simulink model "MDCC"  (R2021b)
settings: Solver=FixedStepDiscrete  StartTime=0.0  StopTime=10.0  FixedStep=0.0001  RelTol=1e-3
model workspace (MATLAB code in the model file):
  | cmdLim = Simulink.Parameter;
  | cmdLim.Value = 15;
  | cmdLim.Description = 'Limit for controlling the maximum surface command angle.';
  | cmdLim.Min = 0;
  | cmdLim.Max = 90;
  | cmdLim.DocUnits = 'deg';
  | 
  | dispGain = Simulink.Parameter;
  | dispGain.Value = 0.75;
  | dispGain.Description = 'Gain applied to the displacement error.';
  | dispGain.Min = 0;
  | dispGain.Max = [];
  | dispGain.DocUnits = 'deg/sec/deg';
  | 
  | dispLim = Simulink.Parameter;
  | dispLim.Value = 30;
  | dispLim.Description = 'Limit for controlling the maximum commanded angle.';
  | dispLim.Min = 0;
  | dispLim.Max = 180;
  | dispLim.DocUnits = 'deg';
  | 
  | intGain = Simulink.Parameter;
  | intGain.Value = 0.5;
  | intGain.Description = 'Gain applied to the integral error.';
  | intGain.Min = 0;
  | intGain.Max = [];
  | intGain.DocUnits = 'deg/sec/deg/sec';
  | 
  | intLim = Simulink.Parameter;
  | intLim.Value = 5;
  | intLim.Description = 'Limit for controlling the maximum commanded angle.';
  | intLim.Min = 0;
  | intLim.Max = 90;
  | intLim.DocUnits = 'deg';
  | 
  | rateGain = Simulink.Parameter;
  | rateGain.Value = 2;
  | rateGain.Description = 'Gain applied to the rate error.';
  | rateGain.Min = 0;
  | rateGain.Max = [];
  | rateGain.DocUnits = 'deg/deg/sec';
  | 
  | rateLim = Simulink.Parameter;
  | rateLim.Value = 6;
  | rateLim.Description = 'Limit for controlling the maximum commanded angle.';
  | rateLim.Min = 0;
  | rateLim.Max = 180;
  | rateLim.DocUnits = 'deg/sec';
  | 
  | hdgGain = Simulink.Parameter;
  | hdgGain.Value = 0.015;
values from neighbouring files (symbols this model uses):
  KfDeadCompen_SetDeltaTime_us = myPackage.Parameter    [DeadCompen.m]
  Ts = 5E-6    (= 5e-06)    [iPMSM_data.m]
  VbDeadComp_SwtUseIsttrDes_flg = myPackage.Parameter    [DeadCompen.m]
  VfDeadCompen_ISttrDdeThdSwt_A = myPackage.Parameter    [DeadCompen.m]
  VfDeadCompen_ISttrIgbtThdSwt_A = myPackage.Parameter    [DeadCompen.m]
  VfDeadCompen_rDdeISttrHi_R = myPackage.Parameter    [DeadCompen.m]
  VfDeadCompen_rDdeISttrLo_R = myPackage.Parameter    [DeadCompen.m]
  VfDeadCompen_rIgbtISttrHi_R = myPackage.Parameter    [DeadCompen.m]
  VfDeadCompen_rIgbtISttrLo_R = myPackage.Parameter    [DeadCompen.m]
  VfDeadCompen_uDdeISttrHi_V = myPackage.Parameter    [DeadCompen.m]
  VfDeadCompen_uDdeISttrLo_V = myPackage.Parameter    [DeadCompen.m]
  VfDeadCompen_uIgbtISttrHi_V = myPackage.Parameter    [DeadCompen.m]
  VfDeadCompen_uIgbtISttrLo_V = myPackage.Parameter    [DeadCompen.m]
undefined symbols (not defined in the file or in its folder): CosTable12bit_Y, GLBCal_GLBCal_Kf_DCLinkOverVolErrThd_V, GLBCal_GLBCal_Kf_DCLinkUnderVolErrThd_V, GLBCal_GLBCal_Kf_EquiLd_NULL, GLBCal_GLBCal_Kf_EquiLq_NULL, GLBCal_GLBCal_Kf_MotorRatedSpeed_rpm, GLBCal_GLBCal_Kf_MotorSpeedHysteresis_Coef, GLBCal_Ke_MotorPolePairsNum_NULL, IoHwAbOpArg_PwmDutyCyclePhU_NULL, IoHwAbOpArg_PwmDutyCyclePhV_NULL, IoHwAbOpArg_PwmDutyCyclePhW_NULL, IoHwAbOpArg_PwmOutputEn, KbMDCC_DeadTimeCompEn_flg, KbMDCC_MCF_flgHarmInIsdqTab11ZR_flg, KbMDCC_MCF_flgHarmInIsdqTab13ZR_flg, KbMDCC_MCF_flgHarmInIsdqTab5ZR_flg, KbMDCC_MCF_flgHarmInIsdqTab7ZR_flg, KbMDCC_MCF_flgHarmInject_flg, KbMDCC_SetEAngleEn_flg, KbMDCC_UdUqFwOmit_flg, KfDeadCompen_CpPeriodTimesT_NULL, KfMDCC_ActiveDischargeIdCurVal_A, KfMDCC_ActiveDischargeIqCurVal_A, KfMDCC_DCLinkVolRate_coef, KfMDCC_DebugEAngleInit_rad, KfMDCC_DebugUalphaVolCmd_V, KfMDCC_DebugUbetaVolCmd_V, KfMDCC_DebugUdCmd_V, KfMDCC_DebugUqCmd_V, KfMDCC_DebugUsCmd_V, KfMDCC_DebugUsRate_V, KfMDCC_IMCResp_NULL, KfMDCC_IMCStab_NULL, KfMDCC_InvParkCpPeriodTimesT_NULL, KfMDCC_MCF_CircAge_NULL, KfMDCC_MCF_flgUse11Harm_flg, KfMDCC_MCF_flgUse13Harm_flg, KfMDCC_MCF_flgUse5Harm_flg, KfMDCC_MCF_flgUse7Harm_flg, KfMDCC_MCF_Harm1113FLParamSpeedThrd_rads, KfMDCC_MCF_Harm57FLParamSpeedThrd_rads, KfMDCC_MCF_HarmcofFltN_NULL, KfMDCC_MCF_HarmCpnAg_NULL, KfMDCC_MCF_HarmfLParaHigh_coef, KfMDCC_MCF_HarmfLParaLow_coef, KfMDCC_MCF_HarmIn1113ZRY_Trq_Nm, KfMDCC_MCF_HarmIn11_SpdLimHigh_rads, KfMDCC_MCF_HarmIn11_SpdLimLow_rads, KfMDCC_MCF_HarmIn11ZRY_Isd_A, KfMDCC_MCF_HarmIn11ZRY_Isq_A, KfMDCC_MCF_HarmIn13_SpdLimHigh_rads, KfMDCC_MCF_HarmIn13_SpdLimLow_rads, KfMDCC_MCF_HarmIn13ZRY_Isd_A, KfMDCC_MCF_HarmIn13ZRY_Isq_A, KfMDCC_MCF_HarmIn57ZRY_Trq_Nm, KfMDCC_MCF_HarmIn5_SpdLimHigh_rads, KfMDCC_MCF_HarmIn5_SpdLimLow_rads, KfMDCC_MCF_HarmIn5ZRY_Isd_A, KfMDCC_MCF_HarmIn5ZRY_Isq_A, KfMDCC_MCF_HarmIn7_SpdLimHigh_rads ... (+47)
libraries: simulink x40, PMSM_Library x3, mcbcontrolslib x1
(part 3 of 8)

== system MDCC/DoCurCtr_sys/MDCC/SVM_Calc/DeadComp_Sys/DeadDuty_Calc ==
  Bus_DutyCompensate : Inport
  CntSctrIs : Inport  Port=2
  Bus Creator : BusCreator  Inputs=7
  Bus Selector : BusSelector  OutputSignals=PwmDuty_0.uDuty,PwmDuty_1.uDuty,PwmDuty_2.uDuty,PwmDuty_3.uDuty,PwmDuty_4.uDuty,PwmDuty_5.uDuty,PwmDuty_fault.uDuty
  Bus Selector1 : BusSelector  OutputSignals=PwmDuty_1.vDuty,PwmDuty_0.vDuty,PwmDuty_2.vDuty,PwmDuty_3.vDuty,PwmDuty_4.vDuty,PwmDuty_5.vDuty,PwmDuty_fault.vDuty
  Bus Selector2 : BusSelector  OutputSignals=PwmDuty_0.wDuty,PwmDuty_1.wDuty,PwmDuty_2.wDuty,PwmDuty_3.wDuty,PwmDuty_4.wDuty,PwmDuty_5.wDuty,PwmDuty_fault.wDuty
  Merge : Merge  Inputs=7
  Merge1 : Merge  Inputs=7
  Merge2 : Merge  Inputs=7
  Switch Case : SwitchCase  CaseConditions={0,1,2,3,4,5}
  Switch Case Action Subsystem : Subsystem  TreatAsAtomicUnit=on
  Switch Case Action Subsystem1 : Subsystem  TreatAsAtomicUnit=on
  Switch Case Action Subsystem2 : Subsystem  TreatAsAtomicUnit=on
  Switch Case Action Subsystem3 : Subsystem  TreatAsAtomicUnit=on
  Switch Case Action Subsystem4 : Subsystem  TreatAsAtomicUnit=on
  Switch Case Action Subsystem5 : Subsystem  TreatAsAtomicUnit=on
  Switch Case Action Subsystem8 : Subsystem  TreatAsAtomicUnit=on
  VfMDSA_DeadCompPwmDutyCyclePhaseU_NULL : Outport
  VfMDSA_DeadCompPwmDutyCyclePhaseV_NULL : Outport  Port=2
  VfMDSA_DeadCompPwmDutyCyclePhaseW_NULL : Outport  Port=3
  wires:
  CntSctrIs/1 -> Switch Case/1
  Switch Case/1 -> [CASE_0]
  Switch Case/2 -> [CASE_1]
  Switch Case/3 -> [CASE_2]
  Switch Case/4 -> [CASE_3]
  Switch Case/5 -> [CASE_4]
  Switch Case/7 -> [default]
  [CASE_0] -> Switch Case Action Subsystem/Action
  [CASE_1] -> Switch Case Action Subsystem1/Action
  [CASE_2] -> Switch Case Action Subsystem2/Action
  [CASE_3] -> Switch Case Action Subsystem3/Action
  [CASE_4] -> Switch Case Action Subsystem4/Action
  [CASE_5] -> Switch Case Action Subsystem5/Action
  [default] -> Switch Case Action Subsystem8/Action
  Switch Case/6 -> [CASE_5]
  Merge/1 -> VfMDSA_DeadCompPwmDutyCyclePhaseU_NULL/1
  Switch Case Action Subsystem/1(PwmDuty) -> Bus Creator/1  "PwmDuty_0"
  Switch Case Action Subsystem1/1(PwmDuty) -> Bus Creator/2  "PwmDuty_1"
  Switch Case Action Subsystem2/1(PwmDuty) -> Bus Creator/3  "PwmDuty_2"
  Switch Case Action Subsystem3/1(PwmDuty) -> Bus Creator/4  "PwmDuty_3"
  Switch Case Action Subsystem4/1(PwmDuty) -> Bus Creator/5  "PwmDuty_4"
  Switch Case Action Subsystem5/1(PwmDuty) -> Bus Creator/6  "PwmDuty_5"
  Switch Case Action Subsystem8/1(PwmDuty) -> Bus Creator/7  "PwmDuty_fault"
  Merge1/1 -> VfMDSA_DeadCompPwmDutyCyclePhaseV_NULL/1
  Merge2/1 -> VfMDSA_DeadCompPwmDutyCyclePhaseW_NULL/1
  Bus Creator/1 -> Bus Selector2/1, Bus Selector1/1, Bus Selector/1
  Bus Selector/1 -> Merge/1  "<uDuty>"
  Bus Selector/2 -> Merge/2  "<uDuty>"
  Bus Selector/3 -> Merge/3  "<uDuty>"
  Bus Selector/4 -> Merge/4  "<uDuty>"
  Bus Selector/5 -> Merge/5  "<uDuty>"
  Bus Selector/6 -> Merge/6  "<uDuty>"
  Bus Selector/7 -> Merge/7  "<uDuty>"
  Bus Selector1/1 -> Merge1/1  "<vDuty>"
  Bus Selector1/2 -> Merge1/2  "<vDuty>"
  Bus Selector1/3 -> Merge1/3  "<vDuty>"
  Bus Selector1/4 -> Merge1/4  "<vDuty>"
  Bus Selector1/5 -> Merge1/5  "<vDuty>"
  Bus Selector1/6 -> Merge1/6  "<vDuty>"
  Bus Selector1/7 -> Merge1/7  "<vDuty>"
  Bus Selector2/1 -> Merge2/1  "<wDuty>"
  Bus Selector2/2 -> Merge2/2  "<wDuty>"
  Bus Selector2/3 -> Merge2/3  "<wDuty>"
  Bus Selector2/4 -> Merge2/4  "<wDuty>"
  Bus Selector2/5 -> Merge2/5  "<wDuty>"
  Bus Selector2/6 -> Merge2/6  "<wDuty>"
  Bus Selector2/7 -> Merge2/7  "<wDuty>"
  Bus_DutyCompensate/1 -> Switch Case Action Subsystem1/1(Bus_DutyCompensate), Switch Case Action Subsystem2/1(Bus_DutyCompensate), Switch Case Action Subsystem3/1(Bus_DutyCompensate), Switch Case Action Subsystem4/1(Bus_DutyCompensate), Switch Case Action Subsystem5/1(Bus_DutyCompensate), Switch Case Action Subsystem8/1("Bus_DutyCorr "), Switch Case Action Subsystem/1(Bus_DutyCompensate)

== system MDCC/DoCurCtr_sys/MDCC/SVM_Calc/DeadComp_Sys/DeadTime_Calc ==
  U_Phase_Dyc : Inport
  V_Phase_Dyc : Inport  Port=2
  W_Phase_Dyc : Inport  Port=3
  iPhase_U : Inport  Port=4
  iPhase_V : Inport  Port=5
  iPhase_W : Inport  Port=6
  uDcLink : Inport  Port=7
  PwmFreq_Hz : Inport  Port=8
  Bus Creator : BusCreator  Inputs=4
  Bus Creator1 : BusCreator  Inputs=3
  DeadTimeDuty_Calc : Subsystem
  DeltaTimeOnOffDuty_Calc : Subsystem
  Tavon_Calc : Subsystem
  Bus_DutyCompensate : Outport
  wires:
  U_Phase_Dyc/1 -> Bus Creator1/1, Tavon_Calc/1(U_Phase_Dyc)  "DutyPhaseU"
  V_Phase_Dyc/1 -> Bus Creator1/2, Tavon_Calc/2(V_Phase_Dyc)  "DutyPhaseV"
  W_Phase_Dyc/1 -> Bus Creator1/3, Tavon_Calc/3(W_Phase_Dyc)  "DutyPhaseW"
  iPhase_U/1 -> DeltaTimeOnOffDuty_Calc/1(iPhase_U), Tavon_Calc/4(iPhase_U)
  iPhase_V/1 -> DeltaTimeOnOffDuty_Calc/2(iPhase_V), Tavon_Calc/5(iPhase_V)
  iPhase_W/1 -> DeltaTimeOnOffDuty_Calc/3(iPhase_W), Tavon_Calc/6(iPhase_W)
  uDcLink/1 -> Tavon_Calc/7(uDcLink)
  PwmFreq_Hz/1 -> DeadTimeDuty_Calc/1(PwmFreq_Hz), DeltaTimeOnOffDuty_Calc/4(PwmFreq_Hz)
  Tavon_Calc/1(Bus_DutyAvon) -> Bus Creator/2  "Bus_DutyAvon"
  DeltaTimeOnOffDuty_Calc/1(Bus_DeltaTimeOnOffDuty) -> Bus Creator/3  "Bus_DeltaTimeOnOffDuty"
  DeadTimeDuty_Calc/1(DeadTimeDuty_NULL) -> Bus Creator/4  "DeadTimeDuty_NULL"
  Bus Creator/1 -> Bus_DutyCompensate/1  "Bus_DutyCompensate"
  Bus Creator1/1 -> Bus Creator/1  "SVM_DutyPhase"

== system MDCC/DoCurCtr_sys/MDCC/SVM_Calc/MDSA/SVM_PU ==
  Ualpha : Inport
  Ubeta : Inport  Port=2
  Add : Sum  Inputs=+-
  Add1 : Sum  Inputs=+-
  Add2 : Sum  Inputs=+-
  Bus Selector : BusSelector  OutputSignals=Tcm1,Tcm2,Tcm3
  Constant : Constant  OutDataTypeStr=single
  Gain : Gain  Gain=2
  Gain1 : Gain  Gain=2
  Gain2 : Gain  Gain=2
  N_Sector_calc : Subsystem
  Saturation : Saturate  UpperLimit=1  LowerLimit=0
  Saturation1 : Saturate  UpperLimit=1  LowerLimit=0
  Saturation2 : Saturate  UpperLimit=1  LowerLimit=0
  Subsystem : Subsystem
  Subsystem1 : Subsystem
  T1_T2_Calc : Subsystem
  Tcm_Calc : Subsystem
  VfMDSA_PwmDutyCyclePhaseU_NULL : Outport  OutMin=0  OutMax=1
  VfMDSA_PwmDutyCyclePhaseV_NULL : Outport  Port=2  OutMin=0  OutMax=1
  VfMDSA_PwmDutyCyclePhaseW_NULL : Outport  Port=3  OutMin=0  OutMax=1
  wires:
  Ualpha/1 -> Subsystem/1(Ualpha), N_Sector_calc/1(Ualpha)
  Ubeta/1 -> Subsystem/2(Ubeta), N_Sector_calc/2(Ubeta)
  N_Sector_calc/1(N_Sector) -> Tcm_Calc/1(N_Sector), T1_T2_Calc/1(N_Sector)
  Subsystem/1(X) -> T1_T2_Calc/2(X)
  Subsystem/2(Y) -> T1_T2_Calc/3(Y)
  Subsystem/3(Z) -> T1_T2_Calc/4(Z)
  Subsystem1/1(Ta) -> Tcm_Calc/2(Ta)
  Subsystem1/2(Tb) -> Tcm_Calc/3(Tb)
  Subsystem1/3(Tc) -> Tcm_Calc/4(Tc)
  Tcm_Calc/1(Bus_CMP) -> Bus Selector/1
  T1_T2_Calc/1(T1) -> Subsystem1/1(T1)
  T1_T2_Calc/2(T2) -> Subsystem1/2(T2)
  Bus Selector/1 -> Gain/1  "<Tcm1>"
  Bus Selector/2 -> Gain1/1  "<Tcm2>"
  Bus Selector/3 -> Gain2/1  "<Tcm3>"
  Constant/1 -> Add2/1, Add1/1, Add/1
  Gain/1 -> Add/2
  Gain1/1 -> Add1/2
  Gain2/1 -> Add2/2
  Add/1 -> Saturation/1
  Add1/1 -> Saturation1/1
  Add2/1 -> Saturation2/1
  Saturation/1 -> VfMDSA_PwmDutyCyclePhaseU_NULL/1
  Saturation1/1 -> VfMDSA_PwmDutyCyclePhaseV_NULL/1
  Saturation2/1 -> VfMDSA_PwmDutyCyclePhaseW_NULL/1

== system MDCC/DoCurCtr_sys/MDCC/SVM_Calc/MDSA/SVPWM ==
  Ualpha_V : Inport
  Ubeta_V : Inport  Port=2
  Ts : Inport  Port=3
  Vdc : Inport  Port=4
  Bus Creator : BusCreator  Inputs=2
  Bus Creator1 : BusCreator  Inputs=2
  Bus Selector : BusSelector  OutputSignals=signal1,signal2,signal3
  Terminator : Terminator
  vIntp_PWMFOC_CalSec : Subsystem  TreatAsAtomicUnit=on  RTWFcnName=vIntp_PWMFOC_CalSec  RTWFileName=vIntp_PWMFOC_CalSec
      settings: RTWFcnNameOpts=User specified  RTWFileNameOpts=User specified
  vIntp_PWMFOC_CalTriCompValue : Subsystem  TreatAsAtomicUnit=on  RTWFcnName=vIntp_PWMFOC_CalTriCompValue  RTWFileName=vIntp_PWMFOC_CalTriCompValue
      settings: RTWFcnNameOpts=User specified  RTWFileNameOpts=User specified
  VfMDSA_PwmDutyCyclePhaseU_NULL : Outport
  VfMDSA_PwmDutyCyclePhaseV_NULL : Outport  Port=2
  VfMDSA_PwmDutyCyclePhaseW_NULL : Outport  Port=3
  wires:
  Bus Selector/3 -> VfMDSA_PwmDutyCyclePhaseW_NULL/1  "<signal3>"
  Bus Selector/2 -> VfMDSA_PwmDutyCyclePhaseV_NULL/1  "<signal2>"
  Bus Selector/1 -> VfMDSA_PwmDutyCyclePhaseU_NULL/1  "<signal1>"
  vIntp_PWMFOC_CalTriCompValue/1(Bus_CMP) -> Bus Selector/1
  vIntp_PWMFOC_CalSec/2(N_VALUE) -> vIntp_PWMFOC_CalTriCompValue/1(N_VALUE_IN)
  vIntp_PWMFOC_CalSec/1(SecValue) -> Terminator/1
  Bus Creator/1 -> vIntp_PWMFOC_CalTriCompValue/2(Bus_UalphaUbeta), vIntp_PWMFOC_CalSec/1(Bus_UalphaUbeta)
  Ualpha_V/1 -> Bus Creator/1  "Ualpha"
  Ubeta_V/1 -> Bus Creator/2  "Ubeta"
  Ts/1 -> Bus Creator1/1  "Ts"
  Vdc/1 -> Bus Creator1/2  "Vdc"
  Bus Creator1/1 -> vIntp_PWMFOC_CalTriCompValue/3(Bus_Ts_Vdc)

== system MDCC/DoCurCtr_sys/MDCC/Simulink Function/Subsystem/If Action Subsystem ==
  In1 : Inport
  Action Port : ActionPort  ActionPortLabel=if(u1 >= u2)
  Constant : Constant  Value=2*pi  OutDataTypeStr=single
  Subtract : Sum  Inputs=+-
  Out1 : Outport
  wires:
  In1/1 -> Subtract/1
  Constant/1 -> Subtract/2
  Subtract/1 -> Out1/1

== system MDCC/DoCurCtr_sys/MDCC/Simulink Function/Subsystem/If Action Subsystem1 ==
  In1 : Inport
  Action Port : ActionPort  ActionPortLabel=elseif(u1 <0)
  Constant : Constant  Value=2*pi  OutDataTypeStr=single
  Subtract : Sum
  Out1 : Outport
  wires:
  In1/1 -> Subtract/1
  Constant/1 -> Subtract/2
  Subtract/1 -> Out1/1

== system MDCC/DoCurCtr_sys/MDCC/Simulink Function/Subsystem/If Action Subsystem2 ==
  In1 : Inport
  Action Port : ActionPort  ActionPortLabel=else
  Out1 : Outport
  wires:
  In1/1 -> Out1/1

== system MDCC/DoCurCtr_sys/MDCC/UdUqCalc_Sys/MDCC_Inverse_Park_Transform/Do_Inverse_Park_Transform ==
  VfMDCC_UdVal_V : Inport
  VfMDCC_UqVal_V : Inport  Port=2
  VfMDCC_SinEAngleNextPWMValue_NULL : Inport  Port=3
  VfMDCC_CosEAngleNextPWMValue_NULL : Inport  Port=4
  Product{,1..3} (4 alike) : Product  RndMeth=Zero
  Subtract : Sum  Inputs=+-
  Subtract1 : Sum
  VfMDCC_VolCmd_alpha_V : Outport
  VfMDCC_VolCmd_beta_V : Outport  Port=2
  wires:
  VfMDCC_UdVal_V/1 -> Product2/1, Product/1
  Product3/1 -> Subtract1/2
  Product2/1 -> Subtract1/1
  Subtract1/1 -> VfMDCC_VolCmd_beta_V/1
  Subtract/1 -> VfMDCC_VolCmd_alpha_V/1
  Product1/1 -> Subtract/2
  VfMDCC_SinEAngleNextPWMValue_NULL/1 -> Product2/2, Product1/2
  VfMDCC_UqVal_V/1 -> Product1/1, Product3/1
  Product/1 -> Subtract/1
  VfMDCC_CosEAngleNextPWMValue_NULL/1 -> Product3/2, Product/2

== system MDCC/DoCurCtr_sys/MDCC/UdUqCalc_Sys/MDCC_MCF_Sys/Clarke1 ==
  VfMDCC_PhaseUCurHarmonic_A : Inport
  VfMDCC_PhaseVCurHarmonic_A : Inport  Port=2
  VfMDCC_PhaseWCurHarmonic_A : Inport  Port=3
  Constant : Constant  Value=0.57735  OutDataTypeStr=single
  Data Type Conversion : DataTypeConversion  OutDataTypeStr=single
  Product : Product
  Subtract : Sum  Inputs=+-
  VfMDCC_AlphaCurHarmonic_A : Outport
  VfMDCC_BetaCurHarmonic_A : Outport  Port=2
  wires:
  Data Type Conversion/1 -> VfMDCC_AlphaCurHarmonic_A/1
  Product/1 -> VfMDCC_BetaCurHarmonic_A/1
  Constant/1 -> Product/2
  Subtract/1 -> Product/1
  VfMDCC_PhaseWCurHarmonic_A/1 -> Subtract/2
  VfMDCC_PhaseVCurHarmonic_A/1 -> Subtract/1
  VfMDCC_PhaseUCurHarmonic_A/1 -> Data Type Conversion/1

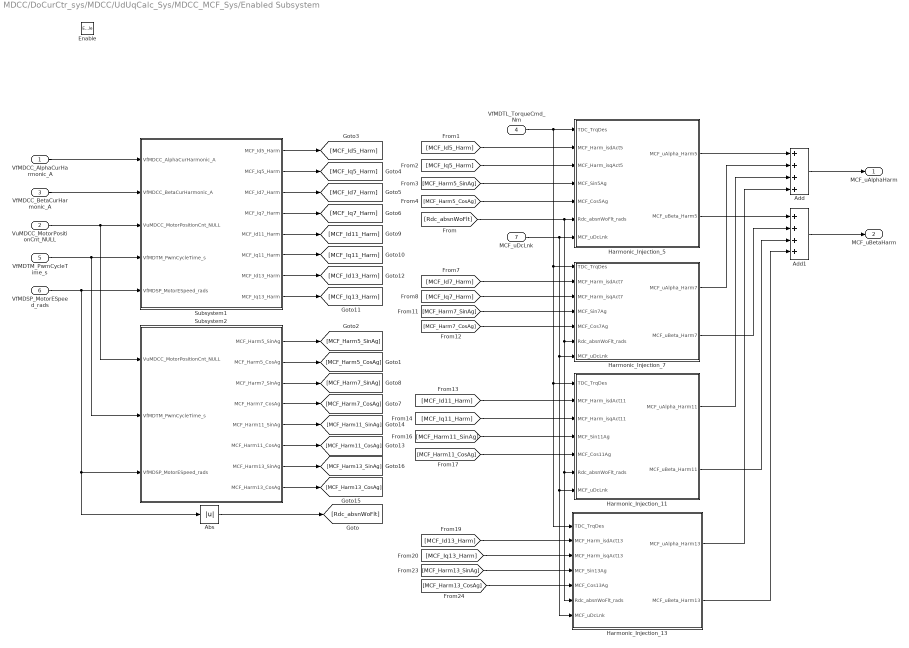
== system MDCC/DoCurCtr_sys/MDCC/UdUqCalc_Sys/MDCC_MCF_Sys/Enabled Subsystem ==
  VfMDCC_AlphaCurHarmonic_A : Inport
  VuMDCC_MotorPositionCnt_NULL : Inport  Port=2
  VfMDCC_BetaCurHarmonic_A : Inport  Port=3
  VfMDTL_TorqueCmd_Nm : Inport  Port=4
  VfMDTM_PwmCycleTime_s : Inport  Port=5
  VfMDSP_MotorESpeed_rads : Inport  Port=6
  MCF_uDcLnk : Inport  Port=7
  Enable : EnablePort
  Abs : Abs
  Add : Sum  Inputs=++++  OutDataTypeStr=single
  Add1 : Sum  Inputs=++++  AccumDataTypeStr=single
  Harmonic_Injection_11 : Subsystem
  Harmonic_Injection_13 : Subsystem
  Harmonic_Injection_5 : Subsystem
  Harmonic_Injection_7 : Subsystem
  Subsystem1 : Subsystem
  Subsystem2 : Subsystem
  MCF_uAlphaHarm : Outport  VectorParamsAs1DForOutWhenUnconnected=off
  MCF_uBetaHarm : Outport  Port=2  VectorParamsAs1DForOutWhenUnconnected=off
  wires:
  VfMDCC_AlphaCurHarmonic_A/1 -> Subsystem1/1(VfMDCC_AlphaCurHarmonic_A)
  VuMDCC_MotorPositionCnt_NULL/1 -> Subsystem2/1(VuMDCC_MotorPositionCnt_NULL), Subsystem1/3(VuMDCC_MotorPositionCnt_NULL)
  VfMDCC_BetaCurHarmonic_A/1 -> Subsystem1/2(VfMDCC_BetaCurHarmonic_A)
  VfMDTM_PwmCycleTime_s/1 -> Subsystem2/2(VfMDTM_PwmCycleTime_s), Subsystem1/4(VfMDTM_PwmCycleTime_s)
  VfMDSP_MotorESpeed_rads/1 -> Abs/1, Subsystem2/3(VfMDSP_MotorESpeed_rads), Subsystem1/5(VfMDSP_MotorESpeed_rads)
  VfMDTL_TorqueCmd_Nm/1 -> Harmonic_Injection_5/1(TDC_TrqDes), Harmonic_Injection_7/1(TDC_TrqDes), Harmonic_Injection_11/1(TDC_TrqDes), Harmonic_Injection_13/1(TDC_TrqDes)
  Subsystem1/1(MCF_Id5_Harm) -> [MCF_Id5_Harm]
  Subsystem1/2(MCF_Iq5_Harm) -> [MCF_Iq5_Harm]
  Subsystem1/3(MCF_Id7_Harm) -> [MCF_Id7_Harm]
  Subsystem1/4(MCF_Iq7_Harm) -> [MCF_Iq7_Harm]
  Subsystem1/5(MCF_Id11_Harm) -> [MCF_Id11_Harm]
  Subsystem1/6(MCF_Iq11_Harm) -> [MCF_Iq11_Harm]
  Subsystem1/7(MCF_Id13_Harm) -> [MCF_Id13_Harm]
  Subsystem1/8(MCF_Iq13_Harm) -> [MCF_Iq13_Harm]
  Subsystem2/1(MCF_Harm5_SinAg) -> [MCF_Harm5_SinAg]
  Subsystem2/2(MCF_Harm5_CosAg) -> [MCF_Harm5_CosAg]
  Subsystem2/3(MCF_Harm7_SinAg) -> [MCF_Harm7_SinAg]
  Subsystem2/4(MCF_Harm7_CosAg) -> [MCF_Harm7_CosAg]
  Subsystem2/5(MCF_Harm11_SinAg) -> [MCF_Harm11_SinAg]
  Subsystem2/6(MCF_Harm11_CosAg) -> [MCF_Harm11_CosAg]
  Subsystem2/7(MCF_Harm13_SinAg) -> [MCF_Harm13_SinAg]
  Subsystem2/8(MCF_Harm13_CosAg) -> [MCF_Harm13_CosAg]
  Abs/1 -> [Rdc_absnWoFlt]
  [MCF_Id5_Harm] -> Harmonic_Injection_5/2(MCF_Harm_isdAct5)
  [MCF_Iq5_Harm] -> Harmonic_Injection_5/3(MCF_Harm_isqAct5)
  [MCF_Harm5_SinAg] -> Harmonic_Injection_5/4(MCF_Sin5Ag)
  [MCF_Harm5_CosAg] -> Harmonic_Injection_5/5(MCF_Cos5Ag)
  [Rdc_absnWoFlt] -> Harmonic_Injection_13/6(Rdc_absnWoFlt_rads), Harmonic_Injection_11/6(Rdc_absnWoFlt_rads), Harmonic_Injection_7/6(Rdc_absnWoFlt_rads), Harmonic_Injection_5/6(Rdc_absnWoFlt_rads)
  MCF_uDcLnk/1 -> Harmonic_Injection_13/7(MCF_uDcLnk), Harmonic_Injection_11/7(MCF_uDcLnk), Harmonic_Injection_7/7(MCF_uDcLnk), Harmonic_Injection_5/7(MCF_uDcLnk)
  [MCF_Id7_Harm] -> Harmonic_Injection_7/2(MCF_Harm_isdAct7)
  [MCF_Iq7_Harm] -> Harmonic_Injection_7/3(MCF_Harm_isqAct7)
  [MCF_Harm7_SinAg] -> Harmonic_Injection_7/4(MCF_Sin7Ag)
  [MCF_Harm7_CosAg] -> Harmonic_Injection_7/5(MCF_Cos7Ag)
  [MCF_Id11_Harm] -> Harmonic_Injection_11/2(MCF_Harm_isdAct11)
  [MCF_Iq11_Harm] -> Harmonic_Injection_11/3(MCF_Harm_isqAct11)
  [MCF_Harm11_SinAg] -> Harmonic_Injection_11/4(MCF_Sin11Ag)
  [MCF_Harm11_CosAg] -> Harmonic_Injection_11/5(MCF_Cos11Ag)
  [MCF_Id13_Harm] -> Harmonic_Injection_13/2(MCF_Harm_isdAct13)
  [MCF_Iq13_Harm] -> Harmonic_Injection_13/3(MCF_Harm_isqAct13)
  [MCF_Harm13_SinAg] -> Harmonic_Injection_13/4(MCF_Sin13Ag)
  [MCF_Harm13_CosAg] -> Harmonic_Injection_13/5(MCF_Cos13Ag)
  Add/1 -> MCF_uAlphaHarm/1
  Harmonic_Injection_5/2(MCF_uBeta_Harm5) -> Add1/1
  Harmonic_Injection_5/1(MCF_uAlpha_Harm5) -> Add/1
  Harmonic_Injection_11/2(MCF_uBeta_Harm11) -> Add1/3
  Add1/1 -> MCF_uBetaHarm/1
  Harmonic_Injection_13/1(MCF_uAlpha_Harm13) -> Add/4
  Harmonic_Injection_7/2(MCF_uBeta_Harm7) -> Add1/2
  Harmonic_Injection_11/1(MCF_uAlpha_Harm11) -> Add/3
  Harmonic_Injection_7/1(MCF_uAlpha_Harm7) -> Add/2
  Harmonic_Injection_13/2(MCF_uBeta_Harm13) -> Add1/4

== system MDCC/DoCurCtr_sys/MDCC/UdUqCalc_Sys/MDCC_MCF_Sys/Subsystem ==
  VfMDSP_PhaseUCurVal_A : Inport  OutDataTypeStr=single
  VfMDSP_PhaseVCurVal_A : Inport  Port=2  OutDataTypeStr=single
  VfMDSP_PhaseWCurVal_A : Inport  Port=3  OutDataTypeStr=single
  VfMDTM_PwmCycleTime_s : Inport  Port=4  OutDataTypeStr=single
  VfMDSP_MotorESpeed_rads : Inport  Port=5  OutDataTypeStr=single
  Add : Sum  Inputs=+-
  Add1 : Sum  Inputs=+-
  Add2 : Sum  Inputs=+-
  iU_SOGI : Subsystem  TreatAsAtomicUnit=on
      settings: RTWSystemCode=Nonreusable function
  iV_SOGI : Subsystem  TreatAsAtomicUnit=on
      settings: RTWSystemCode=Nonreusable function
  iW_SOGI : Subsystem  TreatAsAtomicUnit=on
      settings: RTWSystemCode=Nonreusable function
  VfMDCC_PhaseUCurHarmonic_A : Outport
  VfMDCC_PhaseVCurHarmonic_A : Outport  Port=2
  VfMDCC_PhaseWCurHarmonic_A : Outport  Port=3
  wires:
  iW_SOGI/1(iPhaseBase_A) -> Add2/2
  VfMDSP_PhaseUCurVal_A/1 -> iU_SOGI/1(MCF_iPhase), Add/1
  VfMDSP_MotorESpeed_rads/1 -> iW_SOGI/2(MotorESpeed_rads), iV_SOGI/2(MotorESpeed_rads), iU_SOGI/2(MotorESpeed_rads)
  iU_SOGI/1(iPhaseBase_A) -> Add/2
  VfMDTM_PwmCycleTime_s/1 -> iW_SOGI/3(PwmCycleTime_s), iV_SOGI/3(PwmCycleTime_s), iU_SOGI/3(PwmCycleTime_s)
  VfMDSP_PhaseVCurVal_A/1 -> iV_SOGI/1(MCF_iPhase), Add1/1
  Add1/1 -> VfMDCC_PhaseVCurHarmonic_A/1
  VfMDSP_PhaseWCurVal_A/1 -> iW_SOGI/1(MCF_iPhase), Add2/1
  iV_SOGI/1(iPhaseBase_A) -> Add1/2
  Add/1 -> VfMDCC_PhaseUCurHarmonic_A/1
  Add2/1 -> VfMDCC_PhaseWCurHarmonic_A/1

== system MDCC/DoCurCtr_sys/MDCC/UdUqCalc_Sys/ModDegPwrFacCal/isCal ==
  id : Inport
  iq : Inport  Port=2
  Add : Sum
  Product : Product
  Product1 : Product
  Sqrt : Sqrt  SaturateOnIntegerOverflow=on
  is : Outport
  wires:
  iq/1 -> Product1/2, Product1/1
  id/1 -> Product/2, Product/1
  Product1/1 -> Add/2
  Sqrt/1 -> is/1
  Product/1 -> Add/1
  Add/1 -> Sqrt/1

== system MDCC/DoCurCtr_sys/MDCC/UdUqCalc_Sys/ModDegPwrFacCal/pwrCal ==
  id : Inport
  iq : Inport  Port=2
  ud : Inport  Port=3
  uq : Inport  Port=4
  Add : Sum
  Product : Product
  Product1 : Product
  pwr : Outport
  wires:
  Product/1 -> Add/1
  Product1/1 -> Add/2
  id/1 -> Product/1
  ud/1 -> Product/2
  iq/1 -> Product1/1
  uq/1 -> Product1/2
  Add/1 -> pwr/1

== system MDCC/DoCurCtr_sys/MDCC/UdUqCalc_Sys/ModDegPwrFacCal/usCal ==
  ud : Inport
  uq : Inport  Port=2
  Add : Sum
  Product : Product
  Product1 : Product
  Sqrt : Sqrt  SaturateOnIntegerOverflow=on
  us : Outport
  wires:
  Add/1 -> Sqrt/1
  Product/1 -> Add/1
  Sqrt/1 -> us/1
  Product1/1 -> Add/2
  ud/1 -> Product/1, Product/2
  uq/1 -> Product1/1, Product1/2

== system MDCC/DoCurCtr_sys/MDCC/UdUqCalc_Sys/SelfHeating/Subsystem1 ==
  VfMDTM_SelfHeatingEAngle_NULL : Inport
  VbMDTM_SelfHeatingSinWaveEn_flg : Inport  Port=2
  VbMDSP_McuFSelfheatingMode_flg : Inport  Port=3
  Constant : Constant  Value=uint8(100)
  Constant1 : Constant  Value=KfMDCC_SelfHeatingUdVal_V
  Constant3 : Constant  Value=0  OutDataTypeStr=single
  Constant6 : Constant  Value=KfMDCC_SelfHeatingUdValRate_V
  Merge : Merge
  NOT : Logic  Operator=NOT  IconShape=distinctive  AllPortsSameDT=off  OutDataTypeStr=boolean
  Signal Copy : SignalConversion  OverrideOpt=off
  SinCounter_10ms : Subsystem  TreatAsAtomicUnit=on
      settings: RTWSystemCode=Nonreusable function  RTWFcnNameOpts=Use subsystem name
  Subsystem : Subsystem
  Subsystem1 : Subsystem
  Subsystem2 : Subsystem
  Switch : Switch  Criteria=u2 ~= 0
  VfMDCC_SelfHeatingUdVal_V : Outport
  VbMDCC_SelfHeatingStop_flg : Outport  Port=2
  wires:
  VfMDTM_SelfHeatingEAngle_NULL/1 -> Subsystem2/1(VfMDTM_SelfHeatingEAngle_NULL), Subsystem/1(VfMDTM_SelfHeatingEAngle_NULL)
  VbMDTM_SelfHeatingSinWaveEn_flg/1 -> NOT/1, Subsystem/Enable
  NOT/1 -> Subsystem2/Enable
  Subsystem/1(VfMDTM_SelfHeatingUdVal_V) -> Merge/1
  Subsystem2/1(VfMDTM_SelfHeatingUdVal_V) -> Merge/2
  Merge/1 -> Signal Copy/1  "MDCC_VfMDCC_SelfHeatingUdVal_V"
  Constant6/1 -> Subsystem1/2(rate)
  SinCounter_10ms/1(En) -> Subsystem1/Enable  "En"
  Constant/1 -> SinCounter_10ms/1(CNT)
  Subsystem1/1(VfMDTM_SelfHeatingUdVal_V_Set) -> Subsystem/2(VfMDTM_SelfHeatingUdVal_V_Set), Subsystem2/2(VfMDTM_SelfHeatingUdVal_V_Set)  "VfMDTM_SelfHeatingUdVal_V_Set"
  Subsystem1/2(VbMDCC_SelfHeatingStop_flg) -> VbMDCC_SelfHeatingStop_flg/1
  Constant3/1 -> Switch/3
  Constant1/1 -> Switch/1
  Switch/1 -> Subsystem1/1(set)
  VbMDSP_McuFSelfheatingMode_flg/1 -> Switch/2
  Signal Copy/1 -> VfMDCC_SelfHeatingUdVal_V/1

== system MDCC/DoCurCtr_sys/MDCC/UdUqCalc_Sys/UdUqCalc/IsDQCtl_200us ==
  PIReset : Inport
  TQC_IsdDes : Inport  Port=2
  TQC_IsqDes : Inport  Port=3
  ISM_Isd : Inport  Port=4
  ISM_Isq : Inport  Port=5
  TQC_omSttr : Inport  Port=6
  TQC_dtIsctl_Cc : Inport  Port=7
  TQC_kidq : Inport  Port=8
  TQC_kpd : Inport  Port=9
  TQC_kpq : Inport  Port=10
  TQC_Rv : Inport  Port=11
  TQC_UsqFluxExc : Inport  Port=12
  TQC_uDaMax_Cc : Inport  Port=13
  TQC_uQaMax_Cc : Inport  Port=14
  IsDQCtl_m : MATLAB Function  TreatAsAtomicUnit=on  VariantControl=IsDQCtl_m
      settings: RTWSystemCode=Nonreusable function  RTWFcnNameOpts=Use subsystem name
  TQC_UsdPI : Outport
  TQC_UsqPI : Outport  Port=2
  facIntglDa_Dbg : Outport  Port=3
  facIntglQa_Dbg : Outport  Port=4
  facIntglDaQa_Dbg : Outport  Port=5
  uDaUnlim_Dbg : Outport  Port=6
  uQaUnlim_Dbg : Outport  Port=7
  iDaDes_Dbg : Outport  Port=8
  iQaDes_Dbg : Outport  Port=9

== system MDCC/DoCurCtr_sys/MDCC/UdUqCalc_Sys/UdUqCalc/Subsystem ==
  VfMDSP_MotorAveAbsSpeed_rpm : Inport
  VfMDSP_MotorRs_Ohm : Inport  Port=2
  1-D Lookup Table : Lookup_n-D  NumberOfTableDimensions=1  BreakpointsForDimension1=KfMDCC_SpdIMCResp_rpm  BreakpointsForDimension1DataTypeStr=Inherit: Inherit from 'Breakpoint data'  IndexSearchMethod=Linear search  Table=KfMDCC_IMCResp_NULL  TableDataTypeStr=Inherit: Inherit from 'Table data'  ExtrapMethod=Clip  UseLastTableValue=on  InternalRulePriority=Speed  OutDataTypeStr=Inherit: Inherit from 'Table data'  RndMeth=Simplest
  1-D Lookup Table1 : Lookup_n-D  NumberOfTableDimensions=1  BreakpointsForDimension1=KfMDCC_SpdIMCStab_rpm  BreakpointsForDimension1DataTypeStr=Inherit: Inherit from 'Breakpoint data'  IndexSearchMethod=Linear search  Table=KfMDCC_IMCStab_NULL  TableDataTypeStr=Inherit: Inherit from 'Table data'  ExtrapMethod=Clip  UseLastTableValue=on  InternalRulePriority=Speed  OutDataTypeStr=Inherit: Inherit from 'Table data'  RndMeth=Simplest
  Add : Sum
  Constant : Constant  Value=GLBCal_GLBCal_Kf_EquiLq_NULL
  Constant1 : Constant  Value=GLBCal_GLBCal_Kf_EquiLd_NULL
  Product{,1,4..5} (4 alike) : Product  OutDataTypeStr=single  RndMeth=Round
  VfMDCC_Rv_Ohm : Outport
  KfMDCC_Kidq_NULL : Outport  Port=2
  KfMDCC_Kpd_NULL : Outport  Port=3
  KfMDCC_Kpq_NULL : Outport  Port=4
  wires:
  Product/1 -> VfMDCC_Rv_Ohm/1, Add/1  "VfMDCC_Rv_Ohm"
  VfMDSP_MotorAveAbsSpeed_rpm/1 -> 1-D Lookup Table/1, 1-D Lookup Table1/1
  Constant1/1 -> Product4/2
  [StabAdap] -> Product1/2
  1-D Lookup Table/1 -> [RespScal]  "VfMDCC_RespScal_NULL"
  1-D Lookup Table1/1 -> Product/1
  VfMDSP_MotorRs_Ohm/1 -> Product/2, Add/2
  [RespScal] -> Product4/1
  [RespScal] -> Product5/1
  [RespScal] -> Product1/1
  Constant/1 -> Product5/2
  Product1/1 -> KfMDCC_Kidq_NULL/1  "KfMDCC_Kidq_NULL"
  Add/1 -> [StabAdap]  "VfMDCC_KidqStabAdap_NULL"
  Product5/1 -> KfMDCC_Kpq_NULL/1  "KfMDCC_Kpq_NULL"
  Product4/1 -> KfMDCC_Kpd_NULL/1  "KfMDCC_Kpd_NULL"

== system MDCC/DoCurCtr_sys/MDCC/SVM_Calc/DeadComp_Sys/DeadCur_Calc/Inverse_Clarke_Transform ==
  Alpha : Inport
  Beta : Inport  Port=2
  add_b : Sum  Inputs=-+  RndMeth=Simplest  OutDataTypeStr=Inherit: Same as first input
  add_c : Sum  Inputs=--  RndMeth=Simplest  OutDataTypeStr=Inherit: Same as first input
  one_by_two : Gain  Gain=1/2  RndMeth=Simplest  OutDataTypeStr=Inherit: Same as input
  sqrt3_by_two : Gain  Gain=sqrt(3)/2  RndMeth=Simplest  OutDataTypeStr=Inherit: Same as input
  a : Outport  VectorParamsAs1DForOutWhenUnconnected=off
  b : Outport  Port=2  VectorParamsAs1DForOutWhenUnconnected=off
  c : Outport  Port=3  VectorParamsAs1DForOutWhenUnconnected=off
  wires:
  Beta/1 -> sqrt3_by_two/1
  sqrt3_by_two/1 -> add_c/2, add_b/2
  one_by_two/1 -> add_b/1, add_c/1
  add_c/1 -> c/1
  Alpha/1 -> one_by_two/1, a/1
  add_b/1 -> b/1

== system MDCC/DoCurCtr_sys/MDCC/SVM_Calc/DeadComp_Sys/DeadCur_Calc/IsdqSelect_Calc ==
  IsdDes_A : Inport
  IsqDes_A : Inport  Port=2
  IsdFb_A : Inport  Port=3
  IsqFb_A : Inport  Port=4
  Bus Creator : BusCreator  Inputs=2
  Bus Creator1 : BusCreator  Inputs=2
  Bus Selector : BusSelector  OutputSignals=Isd_A,Isq_A
  Constant : Constant  Value=VbDeadComp_SwtUseIsttrDes_flg
  Switch : Switch  Criteria=u2 ~= 0
  Isd_A : Outport
  Isq_A : Outport  Port=2
  wires:
  Bus Creator1/1 -> Switch/3
  IsqDes_A/1 -> Bus Creator/2  "Isq_A"
  Bus Creator/1 -> Switch/1
  IsqFb_A/1 -> Bus Creator1/2  "Isq_A"
  IsdFb_A/1 -> Bus Creator1/1  "Isd_A"
  Constant/1 -> Switch/2
  IsdDes_A/1 -> Bus Creator/1  "Isd_A"
  Switch/1 -> Bus Selector/1
  Bus Selector/1 -> Isd_A/1  "<Isd_A>"
  Bus Selector/2 -> Isq_A/1  "<Isq_A>"

== system MDCC/DoCurCtr_sys/MDCC/SVM_Calc/DeadComp_Sys/DeadCur_Calc/N_Select_Calc ==
  eMtrSpd_rads : Inport
  eMtrPos_NULL : Inport  Port=2
  VfPwmFreq_Hz : Inport  Port=3
  Isd_A : Inport  Port=4
  Isq_A : Inport  Port=5
  Add : Sum  Inputs=+++
  Constant2 : Constant  Value=2*pi  OutDataTypeStr=single
  Constant3 : Constant  Value=pi/6  OutDataTypeStr=single
  Constant4 : Constant  Value=pi/3  OutDataTypeStr=single
  Data Type Conversion : DataTypeConversion  OutDataTypeStr=uint8
  Data Type Conversion1 : DataTypeConversion  OutDataTypeStr=uint16
  Divide : Product  Inputs=*/
  Gain : Gain  Gain=4095/(2*pi)
  Mod : Math  Operator=mod  SaturateOnIntegerOverflow=on
  Subsystem1 : Subsystem
  Subsystem2 : Subsystem
  PreMtrPos : Outport
  Select_N : Outport  Port=2
  wires:
  Constant3/1 -> Add/3
  Mod/1 -> Divide/1
  Subsystem2/1(PreMtrPos) -> Gain/1, Add/1
  Constant2/1 -> Mod/2
  eMtrPos_NULL/1 -> Subsystem2/2(eMtrPos_NULL)
  Add/1 -> Mod/1
  Subsystem1/1(agIsE) -> Add/2
  Divide/1 -> Data Type Conversion/1
  Constant4/1 -> Divide/2
  Data Type Conversion/1 -> Select_N/1
  Isq_A/1 -> Subsystem1/2(Isq_A)
  Isd_A/1 -> Subsystem1/1(Isd_A)
  VfPwmFreq_Hz/1 -> Subsystem2/3(VfPwmFreq_Hz)
  eMtrSpd_rads/1 -> Subsystem2/1(eMtrSpd_rads)
  Gain/1 -> Data Type Conversion1/1
  Data Type Conversion1/1 -> PreMtrPos/1

== system MDCC/DoCurCtr_sys/MDCC/SVM_Calc/DeadComp_Sys/DeadCur_Calc/SineCosineLookup_Calc ==
  PreMtrPos : Inport
  Cos12bit : LookupNDDirect  NumberOfTableDimensions=1  Table=CosTable12bit_Y  TableDataTypeStr=single
  Sin12bit : LookupNDDirect  NumberOfTableDimensions=1  Table=SinTable12bit_Y  TableDataTypeStr=single
  sin : Outport  VectorParamsAs1DForOutWhenUnconnected=off
  cos : Outport  Port=2  VectorParamsAs1DForOutWhenUnconnected=off
  wires:
  PreMtrPos/1 -> Cos12bit/1, Sin12bit/1
  Cos12bit/1 -> cos/1
  Sin12bit/1 -> sin/1

== system MDCC/DoCurCtr_sys/MDCC/SVM_Calc/DeadComp_Sys/DeadCur_Calc/iPark_Calc ==
  Ds : Inport
  Qs : Inport  Port=2
  sin : Inport  Port=3
  cos : Inport  Port=4
  dcos : Product  RndMeth=Simplest  OutDataTypeStr=Inherit: Same as first input
  dsin : Product  RndMeth=Simplest  OutDataTypeStr=Inherit: Same as first input
  qcos : Product  RndMeth=Simplest  OutDataTypeStr=Inherit: Same as first input
  qsin : Product  RndMeth=Simplest  OutDataTypeStr=Inherit: Same as first input
  sum_alpha : Sum  Inputs=|+-  RndMeth=Simplest  OutDataTypeStr=Inherit: Same as first input
  sum_beta : Sum  Inputs=|++  RndMeth=Simplest  OutDataTypeStr=Inherit: Same as first input
  Alpha : Outport  VectorParamsAs1DForOutWhenUnconnected=off
  Beta : Outport  Port=2  VectorParamsAs1DForOutWhenUnconnected=off
  wires:
  qcos/1 -> sum_beta/1
  Qs/1 -> qsin/1, qcos/1
  dcos/1 -> sum_alpha/1
  sin/1 -> dsin/2, qsin/2
  cos/1 -> qcos/2, dcos/2
  qsin/1 -> sum_alpha/2
  Ds/1 -> dcos/1, dsin/1
  dsin/1 -> sum_beta/2
  sum_beta/1 -> Beta/1
  sum_alpha/1 -> Alpha/1

== system MDCC/DoCurCtr_sys/MDCC/SVM_Calc/DeadComp_Sys/DeadDuty_Calc/Switch Case Action Subsystem ==
  Bus_DutyCompensate : Inport
  Action Port : ActionPort  ActionPortLabel=case [ 0 ]:
  Add : Sum  Inputs=++-
  Add1 : Sum  Inputs=+-+
  Add2 : Sum  Inputs=+-+
  Bus Creator : BusCreator  Inputs=3
  Bus Selector : BusSelector  OutputSignals=Bus_DutyAvon.DeadDutyAvon_U,DeadTimeDuty_NULL,Bus_DeltaTimeOnOffDuty.DeltaTimeOnOffU_NULL
  Bus Selector1 : BusSelector  OutputSignals=Bus_DutyAvon.DeadDutyAvon_V,DeadTimeDuty_NULL,Bus_DeltaTimeOnOffDuty.DeltaTimeOnOffV_NULL
  Bus Selector2 : BusSelector  OutputSignals=Bus_DutyAvon.DeadDutyAvon_W,DeadTimeDuty_NULL,Bus_DeltaTimeOnOffDuty.DeltaTimeOnOffW_NULL
  PwmDuty : Outport
  wires:
  Add/1 -> Bus Creator/1  "uDuty"
  Add1/1 -> Bus Creator/2  "vDuty"
  Add2/1 -> Bus Creator/3  "wDuty"
  Bus Creator/1 -> PwmDuty/1
  Bus_DutyCompensate/1 -> Bus Selector/1, Bus Selector2/1, Bus Selector1/1
  Bus Selector/1 -> Add/1  "<DeadDutyAvon_U>"
  Bus Selector/3 -> Add/3  "<DeltaTimeOnOffU_NULL>"
  Bus Selector1/2 -> Add1/2  "<DeadTimeDuty_NULL>"
  Bus Selector1/1 -> Add1/1  "<DeadDutyAvon_V>"
  Bus Selector2/1 -> Add2/1  "<DeadDutyAvon_W>"
  Bus Selector2/2 -> Add2/2  "<DeadTimeDuty_NULL>"
  Bus Selector/2 -> Add/2  "<DeadTimeDuty_NULL>"
  Bus Selector1/3 -> Add1/3  "<DeltaTimeOnOffV_NULL>"
  Bus Selector2/3 -> Add2/3  "<DeltaTimeOnOffW_NULL>"

== system MDCC/DoCurCtr_sys/MDCC/SVM_Calc/DeadComp_Sys/DeadDuty_Calc/Switch Case Action Subsystem1 ==
  Bus_DutyCompensate : Inport
  Action Port : ActionPort  ActionPortLabel=case [ 1 ]:
  Add : Sum  Inputs=++-
  Add1 : Sum  Inputs=++-
  Add2 : Sum  Inputs=+-+
  Bus Creator : BusCreator  Inputs=3
  Bus Selector : BusSelector  OutputSignals=Bus_DutyAvon.DeadDutyAvon_U,DeadTimeDuty_NULL,Bus_DeltaTimeOnOffDuty.DeltaTimeOnOffU_NULL
  Bus Selector1 : BusSelector  OutputSignals=Bus_DutyAvon.DeadDutyAvon_V,DeadTimeDuty_NULL,Bus_DeltaTimeOnOffDuty.DeltaTimeOnOffV_NULL
  Bus Selector2 : BusSelector  OutputSignals=Bus_DutyAvon.DeadDutyAvon_W,DeadTimeDuty_NULL,Bus_DeltaTimeOnOffDuty.DeltaTimeOnOffW_NULL
  PwmDuty : Outport
  wires:
  Add/1 -> Bus Creator/1  "uDuty"
  Add1/1 -> Bus Creator/2  "vDuty"
  Add2/1 -> Bus Creator/3  "wDuty"
  Bus Creator/1 -> PwmDuty/1
  Bus_DutyCompensate/1 -> Bus Selector/1, Bus Selector2/1, Bus Selector1/1
  Bus Selector/1 -> Add/1  "<DeadDutyAvon_U>"
  Bus Selector/3 -> Add/3  "<DeltaTimeOnOffU_NULL>"
  Bus Selector1/2 -> Add1/2  "<DeadTimeDuty_NULL>"
  Bus Selector1/1 -> Add1/1  "<DeadDutyAvon_V>"
  Bus Selector2/1 -> Add2/1  "<DeadDutyAvon_W>"
  Bus Selector2/2 -> Add2/2  "<DeadTimeDuty_NULL>"
  Bus Selector/2 -> Add/2  "<DeadTimeDuty_NULL>"
  Bus Selector1/3 -> Add1/3  "<DeltaTimeOnOffV_NULL>"
  Bus Selector2/3 -> Add2/3  "<DeltaTimeOnOffW_NULL>"

== system MDCC/DoCurCtr_sys/MDCC/SVM_Calc/DeadComp_Sys/DeadDuty_Calc/Switch Case Action Subsystem2 ==
  Bus_DutyCompensate : Inport
  Action Port : ActionPort  ActionPortLabel=case [ 2 ]:
  Add : Sum  Inputs=+-+
  Add1 : Sum  Inputs=++-
  Add2 : Sum  Inputs=+-+
  Bus Creator : BusCreator  Inputs=3
  Bus Selector : BusSelector  OutputSignals=Bus_DutyAvon.DeadDutyAvon_U,DeadTimeDuty_NULL,Bus_DeltaTimeOnOffDuty.DeltaTimeOnOffU_NULL
  Bus Selector1 : BusSelector  OutputSignals=Bus_DutyAvon.DeadDutyAvon_V,DeadTimeDuty_NULL,Bus_DeltaTimeOnOffDuty.DeltaTimeOnOffV_NULL
  Bus Selector2 : BusSelector  OutputSignals=Bus_DutyAvon.DeadDutyAvon_W,DeadTimeDuty_NULL,Bus_DeltaTimeOnOffDuty.DeltaTimeOnOffW_NULL
  PwmDuty : Outport
  wires:
  Add/1 -> Bus Creator/1  "uDuty"
  Add1/1 -> Bus Creator/2  "vDuty"
  Add2/1 -> Bus Creator/3  "wDuty"
  Bus Creator/1 -> PwmDuty/1
  Bus_DutyCompensate/1 -> Bus Selector/1, Bus Selector2/1, Bus Selector1/1
  Bus Selector/1 -> Add/1  "<DeadDutyAvon_U>"
  Bus Selector/3 -> Add/3  "<DeltaTimeOnOffU_NULL>"
  Bus Selector1/2 -> Add1/2  "<DeadTimeDuty_NULL>"
  Bus Selector1/1 -> Add1/1  "<DeadDutyAvon_V>"
  Bus Selector2/1 -> Add2/1  "<DeadDutyAvon_W>"
  Bus Selector2/2 -> Add2/2  "<DeadTimeDuty_NULL>"
  Bus Selector/2 -> Add/2  "<DeadTimeDuty_NULL>"
  Bus Selector1/3 -> Add1/3  "<DeltaTimeOnOffV_NULL>"
  Bus Selector2/3 -> Add2/3  "<DeltaTimeOnOffW_NULL>"

== system MDCC/DoCurCtr_sys/MDCC/SVM_Calc/DeadComp_Sys/DeadDuty_Calc/Switch Case Action Subsystem3 ==
  Bus_DutyCompensate : Inport
  Action Port : ActionPort  ActionPortLabel=case [ 3 ]:
  Add : Sum  Inputs=+-+
  Add1 : Sum  Inputs=++-
  Add2 : Sum  Inputs=++-
  Bus Creator : BusCreator  Inputs=3
  Bus Selector : BusSelector  OutputSignals=Bus_DutyAvon.DeadDutyAvon_U,DeadTimeDuty_NULL,Bus_DeltaTimeOnOffDuty.DeltaTimeOnOffU_NULL
  Bus Selector1 : BusSelector  OutputSignals=Bus_DutyAvon.DeadDutyAvon_V,DeadTimeDuty_NULL,Bus_DeltaTimeOnOffDuty.DeltaTimeOnOffV_NULL
  Bus Selector2 : BusSelector  OutputSignals=Bus_DutyAvon.DeadDutyAvon_W,DeadTimeDuty_NULL,Bus_DeltaTimeOnOffDuty.DeltaTimeOnOffW_NULL
  PwmDuty : Outport
  wires:
  Add/1 -> Bus Creator/1  "uDuty"
  Add1/1 -> Bus Creator/2  "vDuty"
  Add2/1 -> Bus Creator/3  "wDuty"
  Bus Creator/1 -> PwmDuty/1
  Bus_DutyCompensate/1 -> Bus Selector/1, Bus Selector2/1, Bus Selector1/1
  Bus Selector/1 -> Add/1  "<DeadDutyAvon_U>"
  Bus Selector/3 -> Add/3  "<DeltaTimeOnOffU_NULL>"
  Bus Selector1/2 -> Add1/2  "<DeadTimeDuty_NULL>"
  Bus Selector1/1 -> Add1/1  "<DeadDutyAvon_V>"
  Bus Selector2/1 -> Add2/1  "<DeadDutyAvon_W>"
  Bus Selector2/2 -> Add2/2  "<DeadTimeDuty_NULL>"
  Bus Selector/2 -> Add/2  "<DeadTimeDuty_NULL>"
  Bus Selector1/3 -> Add1/3  "<DeltaTimeOnOffV_NULL>"
  Bus Selector2/3 -> Add2/3  "<DeltaTimeOnOffW_NULL>"

== system MDCC/DoCurCtr_sys/MDCC/SVM_Calc/DeadComp_Sys/DeadDuty_Calc/Switch Case Action Subsystem4 ==
  Bus_DutyCompensate : Inport
  Action Port : ActionPort  ActionPortLabel=case [ 4 ]:
  Add : Sum  Inputs=+-+
  Add1 : Sum  Inputs=+-+
  Add2 : Sum  Inputs=++-
  Bus Creator : BusCreator  Inputs=3
  Bus Selector : BusSelector  OutputSignals=Bus_DutyAvon.DeadDutyAvon_U,DeadTimeDuty_NULL,Bus_DeltaTimeOnOffDuty.DeltaTimeOnOffU_NULL
  Bus Selector1 : BusSelector  OutputSignals=Bus_DutyAvon.DeadDutyAvon_V,DeadTimeDuty_NULL,Bus_DeltaTimeOnOffDuty.DeltaTimeOnOffV_NULL
  Bus Selector2 : BusSelector  OutputSignals=Bus_DutyAvon.DeadDutyAvon_W,DeadTimeDuty_NULL,Bus_DeltaTimeOnOffDuty.DeltaTimeOnOffW_NULL
  PwmDuty : Outport
  wires:
  Add/1 -> Bus Creator/1  "uDuty"
  Add1/1 -> Bus Creator/2  "vDuty"
  Add2/1 -> Bus Creator/3  "wDuty"
  Bus Creator/1 -> PwmDuty/1
  Bus_DutyCompensate/1 -> Bus Selector/1, Bus Selector2/1, Bus Selector1/1
  Bus Selector/1 -> Add/1  "<DeadDutyAvon_U>"
  Bus Selector/3 -> Add/3  "<DeltaTimeOnOffU_NULL>"
  Bus Selector1/2 -> Add1/2  "<DeadTimeDuty_NULL>"
  Bus Selector1/1 -> Add1/1  "<DeadDutyAvon_V>"
  Bus Selector2/1 -> Add2/1  "<DeadDutyAvon_W>"
  Bus Selector2/2 -> Add2/2  "<DeadTimeDuty_NULL>"
  Bus Selector/2 -> Add/2  "<DeadTimeDuty_NULL>"
  Bus Selector1/3 -> Add1/3  "<DeltaTimeOnOffV_NULL>"
  Bus Selector2/3 -> Add2/3  "<DeltaTimeOnOffW_NULL>"

== system MDCC/DoCurCtr_sys/MDCC/SVM_Calc/DeadComp_Sys/DeadDuty_Calc/Switch Case Action Subsystem5 ==
  Bus_DutyCompensate : Inport
  Action Port : ActionPort  ActionPortLabel=case [ 5 ]:
  Add : Sum  Inputs=++-
  Add1 : Sum  Inputs=+-+
  Add2 : Sum  Inputs=++-
  Bus Creator : BusCreator  Inputs=3
  Bus Selector : BusSelector  OutputSignals=Bus_DutyAvon.DeadDutyAvon_U,DeadTimeDuty_NULL,Bus_DeltaTimeOnOffDuty.DeltaTimeOnOffU_NULL
  Bus Selector1 : BusSelector  OutputSignals=Bus_DutyAvon.DeadDutyAvon_V,DeadTimeDuty_NULL,Bus_DeltaTimeOnOffDuty.DeltaTimeOnOffV_NULL
  Bus Selector2 : BusSelector  OutputSignals=Bus_DutyAvon.DeadDutyAvon_W,DeadTimeDuty_NULL,Bus_DeltaTimeOnOffDuty.DeltaTimeOnOffW_NULL
  PwmDuty : Outport
  wires:
  Add/1 -> Bus Creator/1  "uDuty"
  Add1/1 -> Bus Creator/2  "vDuty"
  Add2/1 -> Bus Creator/3  "wDuty"
  Bus Creator/1 -> PwmDuty/1
  Bus_DutyCompensate/1 -> Bus Selector/1, Bus Selector2/1, Bus Selector1/1
  Bus Selector/1 -> Add/1  "<DeadDutyAvon_U>"
  Bus Selector/3 -> Add/3  "<DeltaTimeOnOffU_NULL>"
  Bus Selector1/2 -> Add1/2  "<DeadTimeDuty_NULL>"
  Bus Selector1/1 -> Add1/1  "<DeadDutyAvon_V>"
  Bus Selector2/1 -> Add2/1  "<DeadDutyAvon_W>"
  Bus Selector2/2 -> Add2/2  "<DeadTimeDuty_NULL>"
  Bus Selector/2 -> Add/2  "<DeadTimeDuty_NULL>"
  Bus Selector1/3 -> Add1/3  "<DeltaTimeOnOffV_NULL>"
  Bus Selector2/3 -> Add2/3  "<DeltaTimeOnOffW_NULL>"

== system MDCC/DoCurCtr_sys/MDCC/SVM_Calc/DeadComp_Sys/DeadDuty_Calc/Switch Case Action Subsystem8 ==
  "Bus_DutyCorr " : Inport
  Action Port : ActionPort  ActionPortLabel=default:
  Bus Creator : BusCreator  Inputs=3
  Bus Selector : BusSelector  OutputSignals=SVM_DutyPhase.DutyPhaseU,SVM_DutyPhase.DutyPhaseV,SVM_DutyPhase.DutyPhaseW
  Signal Copy : SignalConversion  OverrideOpt=off
  Signal Copy1 : SignalConversion  OverrideOpt=off
  Signal Copy2 : SignalConversion  OverrideOpt=off
  PwmDuty : Outport
  wires:
  "Bus_DutyCorr "/1 -> Bus Selector/1
  Bus Selector/1 -> Signal Copy/1  "<DutyPhaseU>"
  Signal Copy1/1 -> Bus Creator/2  "vDuty"
  Bus Creator/1 -> PwmDuty/1
  Signal Copy2/1 -> Bus Creator/3  "wDuty"
  Signal Copy/1 -> Bus Creator/1  "uDuty"
  Bus Selector/2 -> Signal Copy1/1  "<DutyPhaseV>"
  Bus Selector/3 -> Signal Copy2/1  "<DutyPhaseW>"

== system MDCC/DoCurCtr_sys/MDCC/SVM_Calc/DeadComp_Sys/DeadTime_Calc/DeadTimeDuty_Calc ==
  PwmFreq_Hz : Inport
  Constant : Constant  Value=KfDeadCompen_SetDeltaTime_us  OutDataTypeStr=single
  Constant1 : Constant  Value=1e6  OutDataTypeStr=single
  Divide2 : Product  Inputs=**/
  DeadTimeDuty_NULL : Outport
  wires:
  Divide2/1 -> DeadTimeDuty_NULL/1  "DeadTimeDuty_NULL"
  Constant/1 -> Divide2/1
  Constant1/1 -> Divide2/3
  PwmFreq_Hz/1 -> Divide2/2

== system MDCC/DoCurCtr_sys/MDCC/SVM_Calc/DeadComp_Sys/DeadTime_Calc/DeltaTimeOnOffDuty_Calc ==
  iPhase_U : Inport
  iPhase_V : Inport  Port=2
  iPhase_W : Inport  Port=3
  PwmFreq_Hz : Inport  Port=4
  1-D Lookup Table1 : Lookup_n-D  Priority=48  NumberOfTableDimensions=1  BreakpointsForDimension1=TableDeadTimeLookUpCur_A  Table=TableDeadTime_us  ExtrapMethod=Clip  UseLastTableValue=on  InternalRulePriority=Speed  RndMeth=Simplest  InputSameDT=on
  1-D Lookup Table2 : Lookup_n-D  Priority=48  NumberOfTableDimensions=1  BreakpointsForDimension1=TableDeadTimeLookUpCur_A  Table=TableDeadTime_us  ExtrapMethod=Clip  UseLastTableValue=on  InternalRulePriority=Speed  RndMeth=Simplest  InputSameDT=on
  1-D Lookup Table3 : Lookup_n-D  Priority=48  NumberOfTableDimensions=1  BreakpointsForDimension1=TableDeadTimeLookUpCur_A  Table=TableDeadTime_us  ExtrapMethod=Clip  UseLastTableValue=on  InternalRulePriority=Speed  RndMeth=Simplest  InputSameDT=on
  Abs : Abs  Priority=39
  Abs1 : Abs  Priority=47
  Abs2 : Abs  Priority=51
  Bus Creator : BusCreator  Inputs=3
  Constant : Constant  Value=1e6  OutDataTypeStr=single
  Divide : Product  Inputs=**/
  Divide1 : Product  Inputs=**/
  Divide2 : Product  Inputs=**/
  Bus_DeltaTimeOnOffDuty : Outport
  wires:
  1-D Lookup Table1/1 -> Divide/1
  1-D Lookup Table3/1 -> Divide2/1
  PwmFreq_Hz/1 -> Divide/2, Divide1/2, Divide2/2
  iPhase_U/1 -> Abs/1
  1-D Lookup Table2/1 -> Divide1/1
  Bus Creator/1 -> Bus_DeltaTimeOnOffDuty/1
  Abs2/1 -> 1-D Lookup Table3/1  "iPhaseAbs"
  iPhase_V/1 -> Abs1/1
  Constant/1 -> Divide/3, Divide1/3, Divide2/3
  Abs1/1 -> 1-D Lookup Table2/1  "iPhaseAbs"
  Abs/1 -> 1-D Lookup Table1/1  "iPhaseAbs"
  Divide1/1 -> Bus Creator/2  "DeltaTimeOnOffV_NULL"
  Divide/1 -> Bus Creator/1  "DeltaTimeOnOffU_NULL"
  Divide2/1 -> Bus Creator/3  "DeltaTimeOnOffW_NULL"
  iPhase_W/1 -> Abs2/1

== system MDCC/DoCurCtr_sys/MDCC/SVM_Calc/DeadComp_Sys/DeadTime_Calc/Tavon_Calc ==
  U_Phase_Dyc : Inport
  V_Phase_Dyc : Inport  Port=2
  W_Phase_Dyc : Inport  Port=3
  iPhase_U : Inport  Port=4
  iPhase_V : Inport  Port=5
  iPhase_W : Inport  Port=6
  uDcLink : Inport  Port=7
  Bus Creator : BusCreator  Inputs=3
  ia : Subsystem  TreatAsAtomicUnit=on
      settings: RTWSystemCode=Nonreusable function
  ib : Subsystem  TreatAsAtomicUnit=on
      settings: RTWSystemCode=Nonreusable function
  ic : Subsystem  TreatAsAtomicUnit=on
      settings: RTWSystemCode=Nonreusable function
  Bus_DutyAvon : Outport
  wires:
  V_Phase_Dyc/1 -> ib/2(Phase_Dyc)
  ib/1("Duty_Avon ") -> Bus Creator/2  "DeadDutyAvon_V"
  U_Phase_Dyc/1 -> ia/2(Phase_Dyc)
  uDcLink/1 -> ic/3(uDcLink), ib/3(uDcLink), ia/3(uDcLink)
  iPhase_V/1 -> ib/1(iPhase)
  ic/1("Duty_Avon ") -> Bus Creator/3  "DeadDutyAvon_W"
  iPhase_W/1 -> ic/1(iPhase)
  W_Phase_Dyc/1 -> ic/2(Phase_Dyc)
  Bus Creator/1 -> Bus_DutyAvon/1  "DutyAvon"
  iPhase_U/1 -> ia/1(iPhase)
  ia/1("Duty_Avon ") -> Bus Creator/1  "DeadDutyAvon_U"

== system MDCC/DoCurCtr_sys/MDCC/SVM_Calc/MDSA/SVM_PU/N_Sector_calc ==
  Ualpha : Inport
  Ubeta : Inport  Port=2
  N_calc : Subsystem
  Uref_Calc : Subsystem
  N_Sector : Outport
  wires:
  Uref_Calc/2(Uref2) -> N_calc/2(Uref2)
  Ualpha/1 -> Uref_Calc/1(Ualpha)
  Ubeta/1 -> Uref_Calc/2(Ubeta)
  Uref_Calc/3(Uref3) -> N_calc/3(Uref3)
  N_calc/1(N_Sector) -> N_Sector/1
  Uref_Calc/1(Uref1) -> N_calc/1(Uref1)

== system MDCC/DoCurCtr_sys/MDCC/SVM_Calc/MDSA/SVM_PU/Subsystem ==
  Ualpha : Inport
  Ubeta : Inport  Port=2
  Add1 : Sum
  Add2 : Sum  Inputs=-+
  ConstanT1 : Constant  Value=2  OutDataTypeStr=single
  ConstanT2 : Constant  Value=sqrt(3)/2  OutDataTypeStr=single
  Constant : Constant  Value=3/2  OutDataTypeStr=single
  ProducT1 : Product
  ProducT2 : Product
  Product : Product
  X : Outport
  Y : Outport  Port=2
  Z : Outport  Port=3
  wires:
  Ualpha/1 -> Product/1
  Constant/1 -> Product/2
  ProducT1/1 -> X/1
  ConstanT1/1 -> ProducT1/2
  Ubeta/1 -> ProducT2/1
  Add1/1 -> Y/1
  Product/1 -> Add2/1, Add1/1
  ProducT2/1 -> ProducT1/1, Add2/2, Add1/2
  ConstanT2/1 -> ProducT2/2
  Add2/1 -> Z/1

== system MDCC/DoCurCtr_sys/MDCC/SVM_Calc/MDSA/SVM_PU/Subsystem1 ==
  T1 : Inport
  T2 : Inport  Port=2
  Add : Sum  Inputs=+--
  Add1 : Sum  Inputs=++-
  Add2 : Sum  Inputs=+++
  Constant : Constant  Value=1/4  OutDataTypeStr=single
  Gain1 : Gain  Gain=1/4
  Gain2 : Gain  Gain=1/4
  Ta : Outport
  Tb : Outport  Port=2
  Tc : Outport  Port=3
  wires:
  T1/1 -> Gain1/1
  T2/1 -> Gain2/1
  Constant/1 -> Add2/1, Add1/1, Add/1
  Add/1 -> Ta/1
  Gain1/1 -> Add2/2, Add1/2, Add/2
  Gain2/1 -> Add1/3, Add2/3, Add/3
  Add1/1 -> Tb/1
  Add2/1 -> Tc/1

== system MDCC/DoCurCtr_sys/MDCC/SVM_Calc/MDSA/SVM_PU/T1_T2_Calc ==
  N_Sector : Inport
  X : Inport  Port=2
  Y : Inport  Port=3
  Z : Inport  Port=4
  Subsystem1 : Subsystem
  Subsystem2 : Subsystem
  T4_T6 : Subsystem  Commented=on
  T1 : Outport
  T2 : Outport  Port=2
  wires:
  X/1 -> Subsystem1/2(X)
  Z/1 -> Subsystem1/4(Z)
  N_Sector/1 -> Subsystem1/1(N_Sector)
  Y/1 -> Subsystem1/3(Y)
  Subsystem1/1(Bus_T4T6) -> Subsystem2/1(Bus_T4T6)
  Subsystem2/1(T1) -> T1/1
  Subsystem2/2(T2) -> T2/1
